simulink model "music"  (R2023b)
settings: Solver=VariableStepAuto  StartTime=0.0  StopTime=10  RelTol=1e-3
values from neighbouring files (symbols this model uses):
  clk = 1000    [GEN_DATA.m]
libraries: hdlsllib x4, dsphdlsigops2 x1, dspvision x1
settings Model: Creator=DELL  LastModifiedBy=DELL

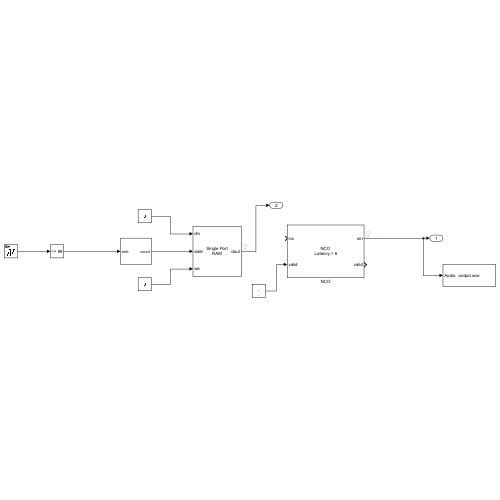
[thumbnail: Simulink's stored preview of the top-level diagram]
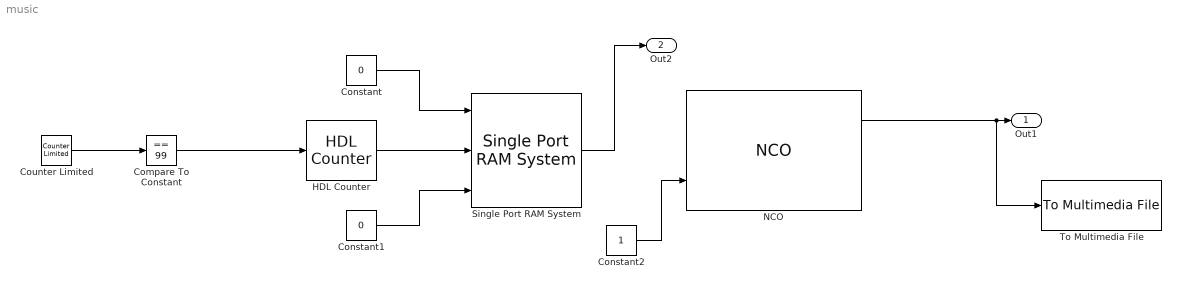
== system music ==
  Compare To Constant : hdlsllib/Logic and Bit Operations/Compare To Constant  relop===  const=99  OutDataTypeStr=boolean
  Constant : Constant  Value=0  OutDataTypeStr=fixdt(1,16,15)  SampleTime=1/clk
  Constant1 : Constant  Value=0  OutDataTypeStr=boolean  SampleTime=1/clk
  Constant2 : Constant  OutDataTypeStr=boolean  SampleTime=1/clk
  Counter Limited : hdlsllib/Sources/Counter Limited  uplimit=99  tsamp=1/clk
  HDL Counter : hdlsllib/Sources/HDL Counter  CountType=Count limited  CountInit=0  CountStep=1  CountMax=6  CountFromType=Initial value  CountFrom=0  CountResetPort=off  CountLoadPort=off  CountEnbPort=on  CountDirPort=off  CountHitOutputPort=off  CountDataType=Unsigned  CountWordLen=8  CountFracLen=0  CountSampTime=1
  NCO : dsphdlsigops2/NCO  PhaseIncrementSource=Input port  PhaseIncrement=100  PhaseOffsetSource=Property  PhaseOffset=0  DitherSource=Property  NumDitherBits=4  SamplesPerFrame=1  LUTCompress=off  ResetAction=off  Waveform=Sine  PhasePort=off  SimulateUsing=Code generation  AccumulatorWL=16  PhaseQuantization=on  NumQuantizerAccumulatorBits=12  OutputDataType=Binary point scaling  OutputWL=16  OutputFL=15
      settings: LibrarySourceBlock=dsphdlsrcs2/NCO
  Single Port RAM System : hdlsllib/HDL RAMs/Single Port RAM System  RAMType=Single port  AsyncRead=off  WriteOutputValue=Old data  RAMInitialValue=fre_word  allowBusInputs=off  WritesHaveOutput=on  NumReads=0  NumWrites=1  SimulateUsing=Code generation
  To Multimedia File : dspvision/To Multimedia File  outputFilename=output.wav  streamSelection=Audio only  videoCompressor=None (uncompressed)  audioCompressor=None (uncompressed)  imagePorts=Separate color signals  fileType=WAV  audioDatatype=16-bit integer  fourcc=RGB  videoQuality=75  mj2000CompFactor=10
      settings: LibrarySourceBlock=audiosinks/To Multimedia File
  Out1 : Outport  VectorParamsAs1DForOutWhenUnconnected=off
  Out2 : Outport  Port=2  VectorParamsAs1DForOutWhenUnconnected=off
  wires:
  Constant/1 -> Single Port RAM System/1
  Constant1/1 -> Single Port RAM System/3
  HDL Counter/1 -> Single Port RAM System/2
  NCO/1 -> To Multimedia File/1, Out1/1
  Compare To Constant/1 -> HDL Counter/1
  Counter Limited/1 -> Compare To Constant/1
  Constant2/1 -> NCO/2
  Single Port RAM System/1 -> Out2/1
